simulink subsystem "CompensadorBateria"  (R2021b)
settings: Solver=VariableStepAuto  StartTime=0.0  StopTime=10.0  RelTol=1e-3
libraries: arduinolib x1
settings Model: Creator=ferna  LastModifiedBy=yo

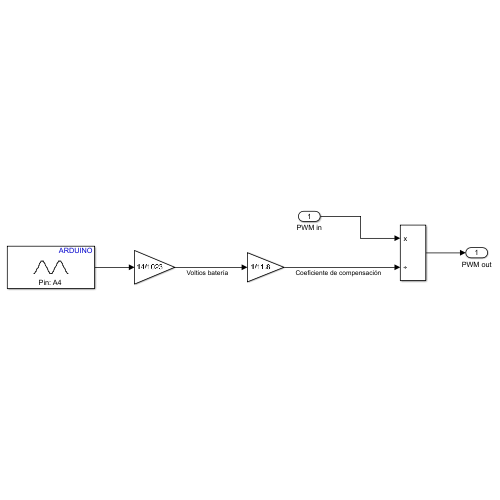
[thumbnail: Simulink's stored preview of the top-level diagram]
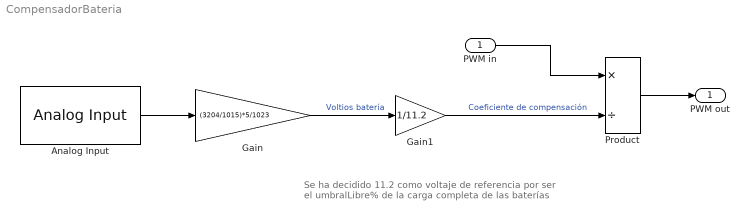
== system CompensadorBateria ==
  note: Se ha decidido 11.2 como voltaje de referencia por ser el umbralLibre% de la carga completa de las baterías
  PWM in : Inport
  Analog Input : arduinolib/Analog Input  pinNumber=0  ReadResultsOnly=off  ConversionTriggerSource=Software  ExternalTriggerType=uint32( 0 )  OutputDataType=uint16  EnableConversionCompleteNotify=off  EnableOuputStatus=off  SampleTime=-1  blockPlatform=arduino
  Gain : Gain  Gain=(3204/1015)*5/1023
  Gain1 : Gain  Gain=1/11.2
  Product : Product  Inputs=*/
  PWM out : Outport
  wires:
  Gain1/1 -> Product/2  "Coeficiente de compensación"
  Gain/1 -> Gain1/1  "Voltios batería"
  Product/1 -> PWM out/1
  PWM in/1 -> Product/1
  Analog Input/1 -> Gain/1
